simulink model "simulink_caso3"  (R2023a)
settings: Solver=VariableStepAuto  StartTime=0.0  StopTime=10.0  RelTol=1e-3
undefined symbols (not defined in the file): A, Aest, B, Best, C, Cest, D, Dest, K00
libraries: simulink x1
settings Model: Creator=Agustin  LastModifiedBy=Agustin

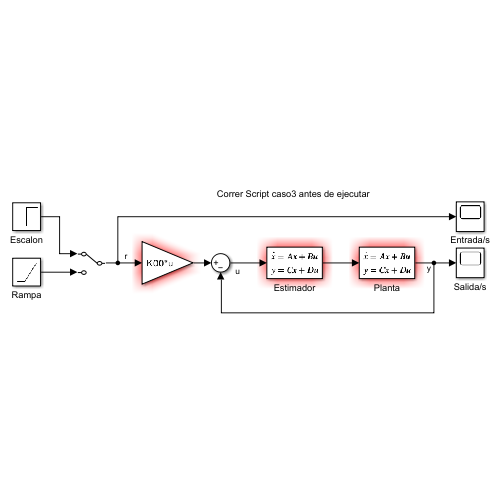
[thumbnail: Simulink's stored preview of the top-level diagram]
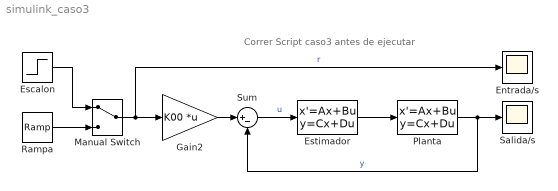
== system simulink_caso3 ==
  note: Correr Script caso3 antes de ejecutar
  Entrada/s : Scope
  Escalon : Step  SampleTime=0
  Estimador : StateSpace  A=Aest  B=Best  C=Cest  D=Dest  InitialCondition=0
  Gain2 : Gain  Gain=K00  Multiplication=Matrix(K*u)
  Manual Switch : ManualSwitch
  Planta : StateSpace  A=A  B=B  C=C  D=D  InitialCondition=0
  Rampa : simulink/Sources/Ramp  slope=1  start=0  InitialOutput=0
  Salida/s : Scope
  Sum : Sum  Inputs=|+-
  wires:
  Escalon/1 -> Manual Switch/1
  Estimador/1 -> Planta/1
  Sum/1 -> Estimador/1  "u"
  Rampa/1 -> Manual Switch/2
  Planta/1 -> Sum/2, Salida/s/1  "y"
  Manual Switch/1 -> Entrada/s/1, Gain2/1  "r"
  Gain2/1 -> Sum/1
